simulink model "Feedback_Linearization"  (R2023a)
settings: Solver=ode1be  StartTime=0.0  StopTime=30  FixedStep=0.1  RelTol=1
settings Model: Creator=suhas  LastModifiedBy=suhas
settings SolverCC: ZeroCrossAlgorithm=Adaptive
settings DebuggingCC: IgnoredZcDiagnostic=none

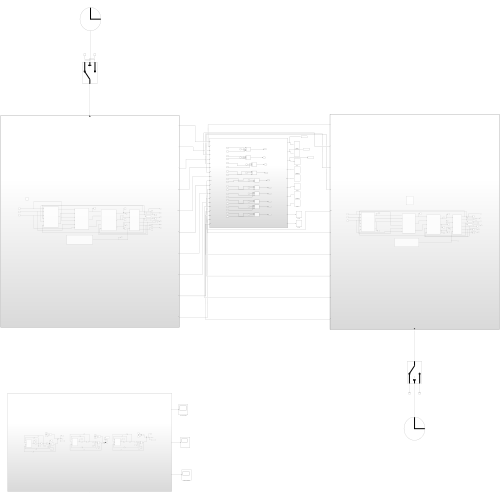
[thumbnail: Simulink's stored preview of the top-level diagram]
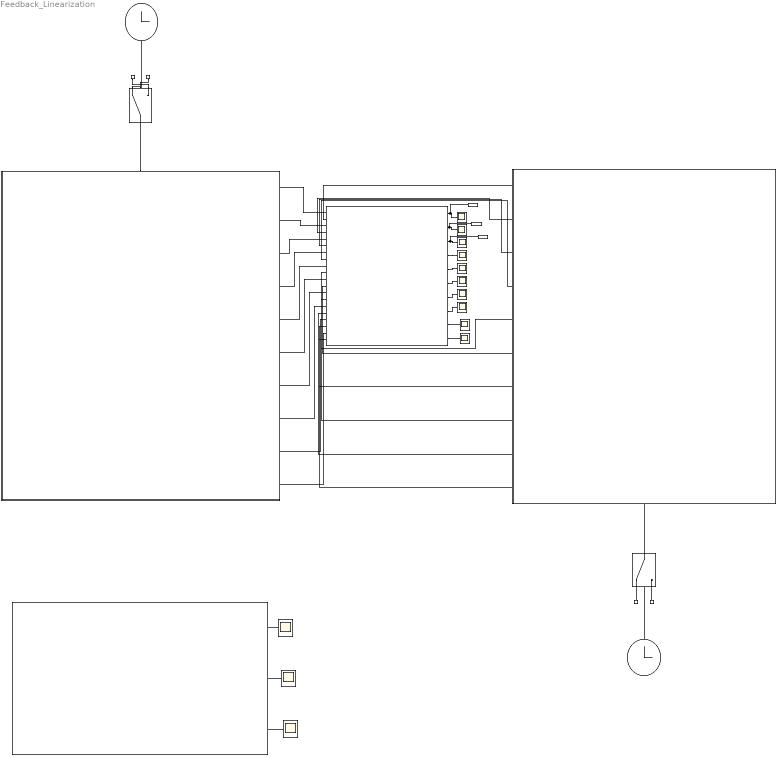
== system Feedback_Linearization ==
  Clock : Clock
  Clock1 : Clock
  Constant : Constant  Value=0
  Constant1 : Constant
  Constant2 : Constant
  Constant3 : Constant  Value=0
  Enabled Subsystem : Subsystem  TreatAsAtomicUnit=on
  Enabled Subsystem1 : Subsystem  TreatAsAtomicUnit=on
  Error Dynamics : Subsystem
  Subsystem : Subsystem
  Switch : Switch  Criteria=u2 > Threshold  Threshold=15  SaturateOnIntegerOverflow=off  InputSameDT=off
  Switch1 : Switch  Criteria=u2 > Threshold  Threshold=15  SaturateOnIntegerOverflow=off  InputSameDT=off
  To Workspace : ToWorkspace  VariableName=x  SaveFormat=Timeseries  SampleTime=-1
  To Workspace1 : ToWorkspace  VariableName=y  SaveFormat=Timeseries  SampleTime=-1
  To Workspace2 : ToWorkspace  VariableName=z  SaveFormat=Timeseries  SampleTime=-1
  X from  Error Dynamics : Scope
  Y from Error Dynamics : Scope
  Z from Error Dynamics : Scope
  phi scope : Scope
  psi scope : Scope
  theta scope : Scope
  u1 scope : Scope
  u2 scope : Scope
  u3 scope : Scope
  u4 scope : Scope
  x scope : Scope
  y scope : Scope
  z scope : Scope
  wires:
  Clock1/1 -> Switch1/2
  Constant3/1 -> Switch1/3
  Clock/1 -> Switch/2
  Constant1/1 -> Switch/3
  Constant2/1 -> Switch1/1
  Constant/1 -> Switch/1
  Switch1/1 -> Enabled Subsystem1/Enable
  Switch/1 -> Enabled Subsystem/Enable
  Enabled Subsystem/1(x) -> Subsystem/1(x1)
  Enabled Subsystem/2(y) -> Subsystem/3(y1)
  Enabled Subsystem/3(z) -> Subsystem/5(z1)
  Enabled Subsystem/4(phi) -> Subsystem/7(phi1)
  Enabled Subsystem/5(theta) -> Subsystem/9(theta1)
  Enabled Subsystem/6(psi) -> Subsystem/11(psi 1)
  Enabled Subsystem/7(u1) -> Subsystem/13(u11)
  Enabled Subsystem/8(u2) -> Subsystem/15(u21)
  Enabled Subsystem/9(u3) -> Subsystem/17(u31)
  Enabled Subsystem/10(u4) -> Subsystem/19(u41)
  Enabled Subsystem1/1(x) -> Subsystem/2(x2)
  Enabled Subsystem1/2(y) -> Subsystem/4(y2)
  Enabled Subsystem1/3(z) -> Subsystem/6(z2)
  Enabled Subsystem1/5(theta) -> Subsystem/10(theta2)
  Enabled Subsystem1/4(phi) -> Subsystem/8(phi2)
  Enabled Subsystem1/6(psi) -> Subsystem/12(psi 2)
  Enabled Subsystem1/8(u1) -> Subsystem/14(u12)
  Enabled Subsystem1/9(u2) -> Subsystem/16(u22)
  Enabled Subsystem1/10(u3) -> Subsystem/18(u32)
  Enabled Subsystem1/7(u4) -> Subsystem/20(u42)
  Subsystem/1(x) -> To Workspace/1, x scope/1
  Subsystem/2(y) -> To Workspace1/1, y scope/1
  Subsystem/3(z) -> To Workspace2/1, z scope/1
  Subsystem/4(phi) -> phi scope/1
  Subsystem/5(theta) -> theta scope/1
  Subsystem/6(psi) -> psi scope/1
  Subsystem/7(u1) -> u1 scope/1
  Subsystem/8(u2) -> u2 scope/1
  Subsystem/9(u3) -> u3 scope/1
  Subsystem/10(u4) -> u4 scope/1
  Error Dynamics/1(x) -> X from  Error Dynamics/1
  Error Dynamics/2(y) -> Y from Error Dynamics/1
  Error Dynamics/3(z) -> Z from Error Dynamics/1

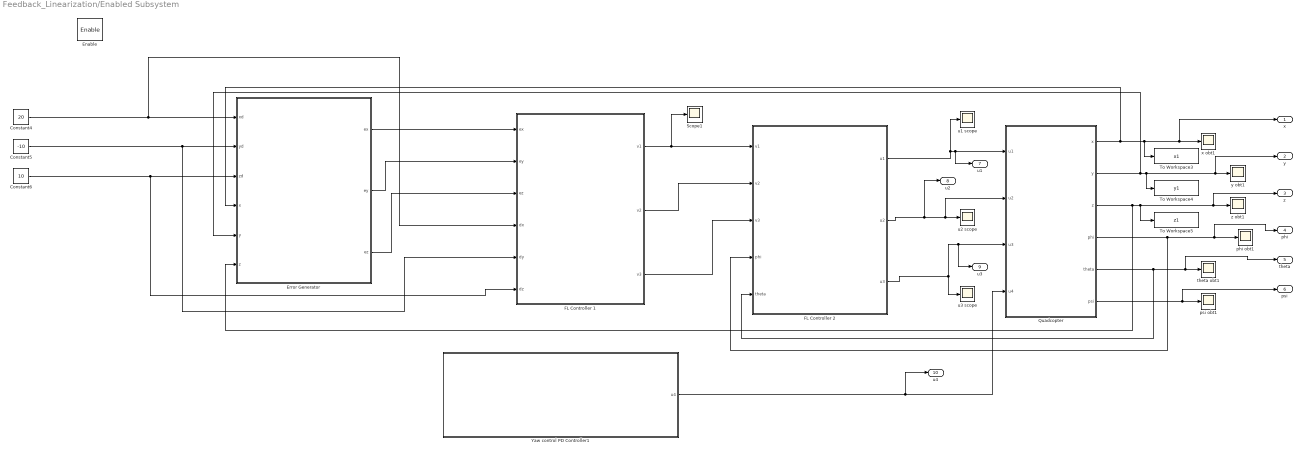
== system Feedback_Linearization/Enabled Subsystem ==
  Enable : EnablePort
  Constant4 : Constant  Value=20
  Constant5 : Constant  Value=-10
  Constant6 : Constant  Value=10
  Error Generator : Subsystem
  FL Controller 1 : Subsystem
  "FL Controller 2 " : Subsystem
  "Quadcopter " : Subsystem
  Scope1 : Scope
  To Workspace3 : ToWorkspace  VariableName=x1  SaveFormat=Timeseries  SampleTime=-1
  To Workspace4 : ToWorkspace  VariableName=y1  SaveFormat=Timeseries  SampleTime=-1
  To Workspace5 : ToWorkspace  VariableName=z1  SaveFormat=Timeseries  SampleTime=-1
  Yaw control PD Controller1 : Subsystem
  phi obt1 : Scope
  psi obt1 : Scope
  theta obt1 : Scope
  u1 scope : Scope
  u2 scope : Scope
  u3 scope : Scope
  x obt1 : Scope
  y obt1 : Scope
  z obt1 : Scope
  x : Outport
  y : Outport  Port=2
  z : Outport  Port=3
  phi : Outport  Port=4
  theta : Outport  Port=5
  psi : Outport  Port=6
  u1 : Outport  Port=7
  u2 : Outport  Port=8
  u3 : Outport  Port=9
  u4 : Outport  Port=10
  wires:
  Error Generator/3(ez) -> FL Controller 1/3(ez)
  "Quadcopter "/1(x) -> Error Generator/4(x), To Workspace3/1, x/1, x obt1/1
  FL Controller 1/2(v2) -> "FL Controller 2 "/2(v2)
  FL Controller 1/1(v1) -> Scope1/1, "FL Controller 2 "/1(v1)
  FL Controller 1/3(v3) -> "FL Controller 2 "/3(v3)
  "Quadcopter "/4(phi) -> "FL Controller 2 "/4(phi), phi/1, phi obt1/1
  "FL Controller 2 "/3(u3) -> u3 scope/1, u3/1, "Quadcopter "/3(u3)
  Error Generator/2(ey) -> FL Controller 1/2(ey)
  Constant4/1 -> FL Controller 1/4(dx), Error Generator/1(xd)
  "Quadcopter "/2(y) -> Error Generator/5(y), To Workspace4/1, y/1, y obt1/1
  "Quadcopter "/6(psi) -> psi/1, psi obt1/1
  Error Generator/1(ex) -> FL Controller 1/1(ex)
  "FL Controller 2 "/1(u1) -> u1 scope/1, u1/1, "Quadcopter "/1(u1)
  Constant6/1 -> FL Controller 1/6(dz), Error Generator/3(zd)
  Yaw control PD Controller1/1(u4) -> u4/1, "Quadcopter "/4(u4)
  Constant5/1 -> FL Controller 1/5(dy), Error Generator/2(yd)
  "FL Controller 2 "/2(u2) -> u2/1, "Quadcopter "/2(u2), u2 scope/1
  "Quadcopter "/5(theta) -> "FL Controller 2 "/5(theta), theta/1, theta obt1/1
  "Quadcopter "/3(z) -> Error Generator/6(z), To Workspace5/1, z/1, z obt1/1

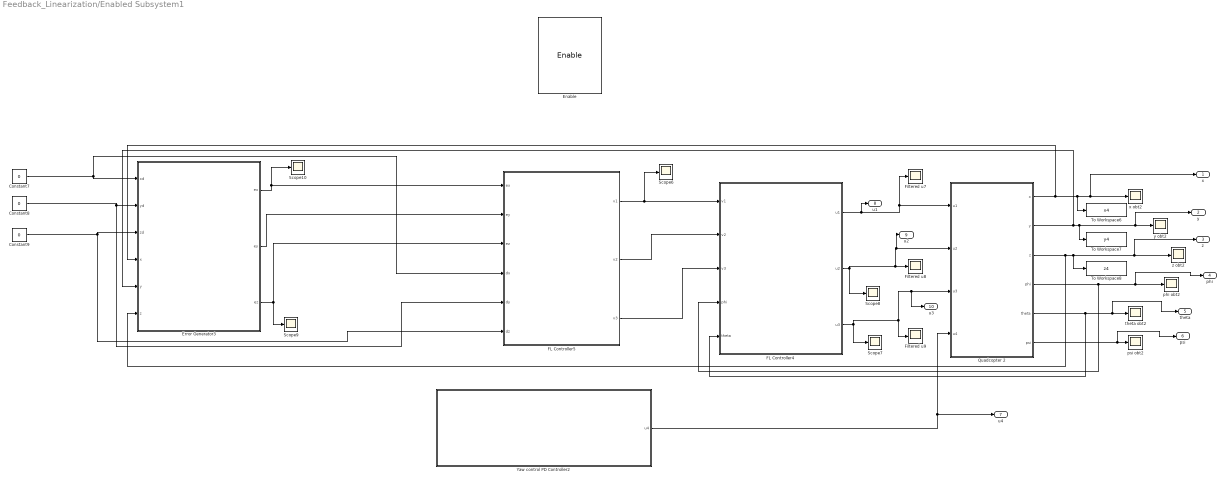
== system Feedback_Linearization/Enabled Subsystem1 ==
  Enable : EnablePort
  Constant7 : Constant  Value=0
  Constant8 : Constant  Value=0
  Constant9 : Constant  Value=0
  Error Generator3 : Subsystem
  FL Controller4 : Subsystem
  FL Controller5 : Subsystem
  Filtered u7 : Scope
  Filtered u8 : Scope
  Filtered u9 : Scope
  Quadcopter 2 : Subsystem
  Scope{6..10} (5 alike) : Scope
  To Workspace6 : ToWorkspace  VariableName=x4  SaveFormat=Timeseries  SampleTime=-1
  To Workspace7 : ToWorkspace  VariableName=y4  SaveFormat=Timeseries  SampleTime=-1
  To Workspace8 : ToWorkspace  VariableName=z4  SaveFormat=Timeseries  SampleTime=-1
  Yaw control PD Controller2 : Subsystem
  phi obt2 : Scope
  psi obt2 : Scope
  theta obt2 : Scope
  x obt2 : Scope
  y obt2 : Scope
  z obt2 : Scope
  x : Outport
  y : Outport  Port=2
  z : Outport  Port=3
  phi : Outport  Port=4
  theta : Outport  Port=5
  psi : Outport  Port=6
  u4 : Outport  Port=7
  u1 : Outport  Port=8
  u2 : Outport  Port=9
  u3 : Outport  Port=10
  wires:
  Quadcopter 2/1(x) -> Error Generator3/4(x), To Workspace6/1, x/1, x obt2/1
  FL Controller5/3(v3) -> FL Controller4/3(v3)
  Quadcopter 2/3(z) -> Error Generator3/6(z), To Workspace8/1, z obt2/1, z/1
  Quadcopter 2/4(phi) -> FL Controller4/4(phi), phi/1, phi obt2/1
  Constant8/1 -> FL Controller5/5(dy), Error Generator3/2(yd)
  Quadcopter 2/5(theta) -> FL Controller4/5(theta), theta/1, theta obt2/1
  FL Controller5/1(v1) -> Scope6/1, FL Controller4/1(v1)
  FL Controller4/3(u3) -> Filtered u9/1, u3/1, Quadcopter 2/3(u3), Scope7/1
  Constant7/1 -> FL Controller5/4(dx), Error Generator3/1(xd)
  Error Generator3/2(ey) -> FL Controller5/2(ey)
  FL Controller4/1(u1) -> u1/1, Filtered u7/1, Quadcopter 2/1(u1)
  FL Controller5/2(v2) -> FL Controller4/2(v2)
  Error Generator3/1(ex) -> Scope10/1, FL Controller5/1(ex)
  Error Generator3/3(ez) -> FL Controller5/3(ez), Scope9/1
  Yaw control PD Controller2/1(u4) -> u4/1, Quadcopter 2/4(u4)
  Constant9/1 -> Error Generator3/3(zd), FL Controller5/6(dz)
  Quadcopter 2/6(psi) -> psi/1, psi obt2/1
  Quadcopter 2/2(y) -> Error Generator3/5(y), To Workspace7/1, y/1, y obt2/1
  FL Controller4/2(u2) -> u2/1, Quadcopter 2/2(u2), Filtered u8/1, Scope8/1

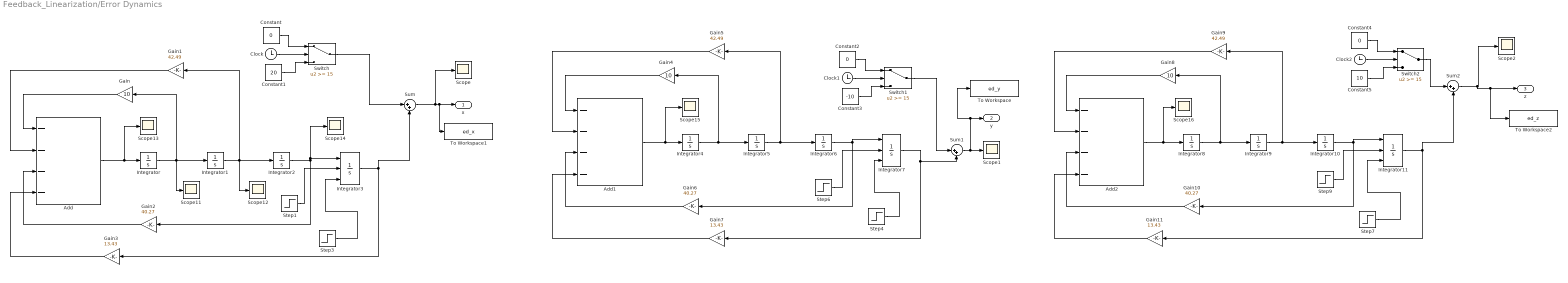
== system Feedback_Linearization/Error Dynamics ==
  Add : Sum  Inputs=----
  Add1 : Sum  Inputs=----
  Add2 : Sum  Inputs=----
  Clock : Clock
  Clock1 : Clock
  Clock2 : Clock
  Constant : Constant  Value=0
  Constant1 : Constant  Value=20
  Constant2 : Constant  Value=0
  Constant3 : Constant  Value=-10
  Constant4 : Constant  Value=0
  Constant5 : Constant  Value=10
  Gain : Gain  Gain=10
  Gain1 : Gain  Gain=42.49
  Gain10 : Gain  Gain=40.27
  Gain11 : Gain  Gain=13.43
  Gain2 : Gain  Gain=40.27
  Gain3 : Gain  Gain=13.43
  Gain4 : Gain  Gain=10
  Gain5 : Gain  Gain=42.49
  Gain6 : Gain  Gain=40.27
  Gain7 : Gain  Gain=13.43
  Gain8 : Gain  Gain=10
  Gain9 : Gain  Gain=42.49
  Integrator{,1..2,4..6,8..10} (9 alike) : Integrator
  Integrator11 : Integrator  ExternalReset=rising  InitialConditionSource=external
  Integrator3 : Integrator  ExternalReset=rising  InitialConditionSource=external
  Integrator7 : Integrator  ExternalReset=rising  InitialConditionSource=external
  Scope{,1..2,11..16} (9 alike) : Scope
  Step1 : Step  Time=15  SampleTime=0
  Step3 : Step  Time=15  Before=-10  After=20  SampleTime=0
  Step4 : Step  Time=15  Before=20  After=-10  SampleTime=0
  Step6 : Step  Time=15  SampleTime=0
  Step7 : Step  Time=15  Before=10  After=10  SampleTime=0
  Step9 : Step  Time=15  SampleTime=0
  Sum : Sum  Inputs=|++
  Sum1 : Sum  Inputs=|++
  Sum2 : Sum  Inputs=|++
  Switch : Switch  Threshold=15  SaturateOnIntegerOverflow=off  InputSameDT=off
  Switch1 : Switch  Threshold=15  SaturateOnIntegerOverflow=off  InputSameDT=off
  Switch2 : Switch  Threshold=15  SaturateOnIntegerOverflow=off  InputSameDT=off
  To Workspace : ToWorkspace  VariableName=ed_y  SaveFormat=Timeseries  SampleTime=-1
  To Workspace1 : ToWorkspace  VariableName=ed_x  SaveFormat=Timeseries  SampleTime=-1
  To Workspace2 : ToWorkspace  VariableName=ed_z  SaveFormat=Timeseries  SampleTime=-1
  x : Outport
  y : Outport  Port=2
  z : Outport  Port=3
  wires:
  Integrator/1 -> Scope11/1, Gain/1, Integrator1/1
  Integrator1/1 -> Scope12/1, Gain1/1, Integrator2/1
  Integrator2/1 -> Scope14/1, Integrator3/1, Gain2/1
  Integrator3/1 -> Sum/2, Gain3/1
  Gain/1 -> Add/1
  Gain1/1 -> Add/2
  Gain2/1 -> Add/3
  Gain3/1 -> Add/4
  Step3/1 -> Integrator3/3
  Switch/1 -> Sum/1
  Sum/1 -> To Workspace1/1, x/1, Scope/1
  Switch1/1 -> Sum1/1
  Gain5/1 -> Add1/2
  Gain4/1 -> Add1/1
  Sum1/1 -> To Workspace/1, y/1, Scope1/1
  Gain7/1 -> Add1/4
  Gain6/1 -> Add1/3
  Switch2/1 -> Sum2/1
  Gain9/1 -> Add2/2
  Gain8/1 -> Add2/1
  Integrator9/1 -> Gain9/1, Integrator10/1
  Gain11/1 -> Add2/4
  Integrator10/1 -> Gain10/1, Integrator11/1
  Gain10/1 -> Add2/3
  Sum2/1 -> To Workspace2/1, z/1, Scope2/1
  Add/1 -> Scope13/1, Integrator/1
  Add1/1 -> Scope15/1, Integrator4/1
  Step4/1 -> Integrator7/3
  Step7/1 -> Integrator11/3
  Add2/1 -> Scope16/1, Integrator8/1
  Step9/1 -> Integrator11/2
  Step6/1 -> Integrator7/2
  Step1/1 -> Integrator3/2
  Integrator7/1 -> Gain7/1, Sum1/2
  Integrator6/1 -> Gain6/1, Integrator7/1
  Integrator5/1 -> Gain5/1, Integrator6/1
  Integrator4/1 -> Gain4/1, Integrator5/1
  Integrator8/1 -> Gain8/1, Integrator9/1
  Integrator11/1 -> Sum2/2, Gain11/1
  Clock/1 -> Switch/2
  Constant/1 -> Switch/1
  Constant1/1 -> Switch/3
  Constant2/1 -> Switch1/1
  Constant3/1 -> Switch1/3
  Clock1/1 -> Switch1/2
  Constant4/1 -> Switch2/1
  Constant5/1 -> Switch2/3
  Clock2/1 -> Switch2/2

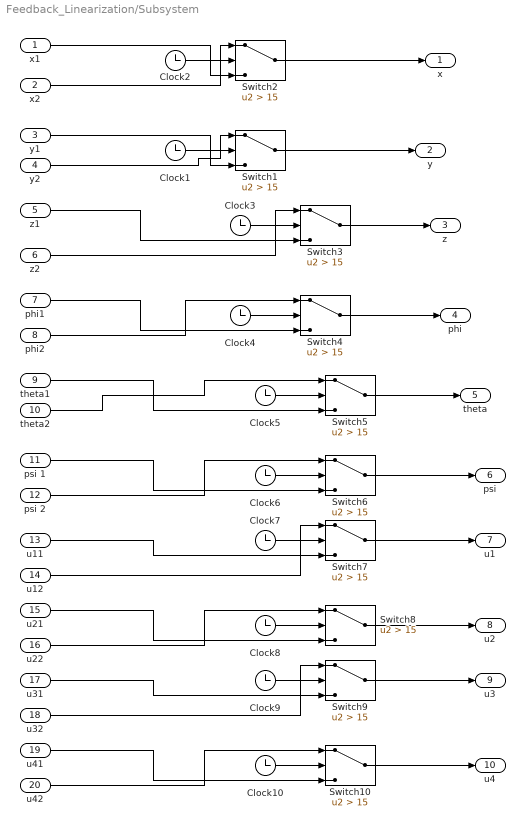
== system Feedback_Linearization/Subsystem ==
  x1 : Inport
  x2 : Inport  Port=2
  y1 : Inport  Port=3
  y2 : Inport  Port=4
  z1 : Inport  Port=5
  z2 : Inport  Port=6
  phi1 : Inport  Port=7
  phi2 : Inport  Port=8
  theta1 : Inport  Port=9
  theta2 : Inport  Port=10
  psi 1 : Inport  Port=11
  psi 2 : Inport  Port=12
  u11 : Inport  Port=13
  u12 : Inport  Port=14
  u21 : Inport  Port=15
  u22 : Inport  Port=16
  u31 : Inport  Port=17
  u32 : Inport  Port=18
  u41 : Inport  Port=19
  u42 : Inport  Port=20
  Clock{1..10} (10 alike) : Clock
  Switch{1..10} (10 alike) : Switch  Criteria=u2 > Threshold  Threshold=15  SaturateOnIntegerOverflow=off  InputSameDT=off
  x : Outport
  y : Outport  Port=2
  z : Outport  Port=3
  phi : Outport  Port=4
  theta : Outport  Port=5
  psi : Outport  Port=6
  u1 : Outport  Port=7
  u2 : Outport  Port=8
  u3 : Outport  Port=9
  u4 : Outport  Port=10
  wires:
  Clock2/1 -> Switch2/2
  x1/1 -> Switch2/3
  x2/1 -> Switch2/1
  y2/1 -> Switch1/1
  Clock1/1 -> Switch1/2
  y1/1 -> Switch1/3
  z2/1 -> Switch3/1
  Clock3/1 -> Switch3/2
  z1/1 -> Switch3/3
  phi2/1 -> Switch4/1
  Clock4/1 -> Switch4/2
  phi1/1 -> Switch4/3
  theta2/1 -> Switch5/1
  Clock5/1 -> Switch5/2
  theta1/1 -> Switch5/3
  psi 2/1 -> Switch6/1
  Clock6/1 -> Switch6/2
  psi 1/1 -> Switch6/3
  u12/1 -> Switch7/1
  Clock7/1 -> Switch7/2
  u11/1 -> Switch7/3
  u22/1 -> Switch8/1
  Clock8/1 -> Switch8/2
  u21/1 -> Switch8/3
  u32/1 -> Switch9/1
  Clock9/1 -> Switch9/2
  u31/1 -> Switch9/3
  u42/1 -> Switch10/1
  Clock10/1 -> Switch10/2
  u41/1 -> Switch10/3
  Switch2/1 -> x/1
  Switch1/1 -> y/1
  Switch3/1 -> z/1
  Switch4/1 -> phi/1
  Switch5/1 -> theta/1
  Switch6/1 -> psi/1
  Switch7/1 -> u1/1
  Switch8/1 -> u2/1
  Switch9/1 -> u3/1
  Switch10/1 -> u4/1

== system Feedback_Linearization/Enabled Subsystem/Error Generator ==
  xd : Inport
  yd : Inport  Port=2
  zd : Inport  Port=3
  x : Inport  Port=4
  y : Inport  Port=5
  z : Inport  Port=6
  Subtract : Sum  Inputs=+-
  Subtract1 : Sum  Inputs=+-
  Subtract2 : Sum  Inputs=+-
  ex : Outport
  ey : Outport  Port=2
  ez : Outport  Port=3
  wires:
  xd/1 -> Subtract/2
  x/1 -> Subtract/1
  Subtract/1 -> ex/1
  yd/1 -> Subtract1/2
  y/1 -> Subtract1/1
  z/1 -> Subtract2/1
  zd/1 -> Subtract2/2
  Subtract1/1 -> ey/1
  Subtract2/1 -> ez/1

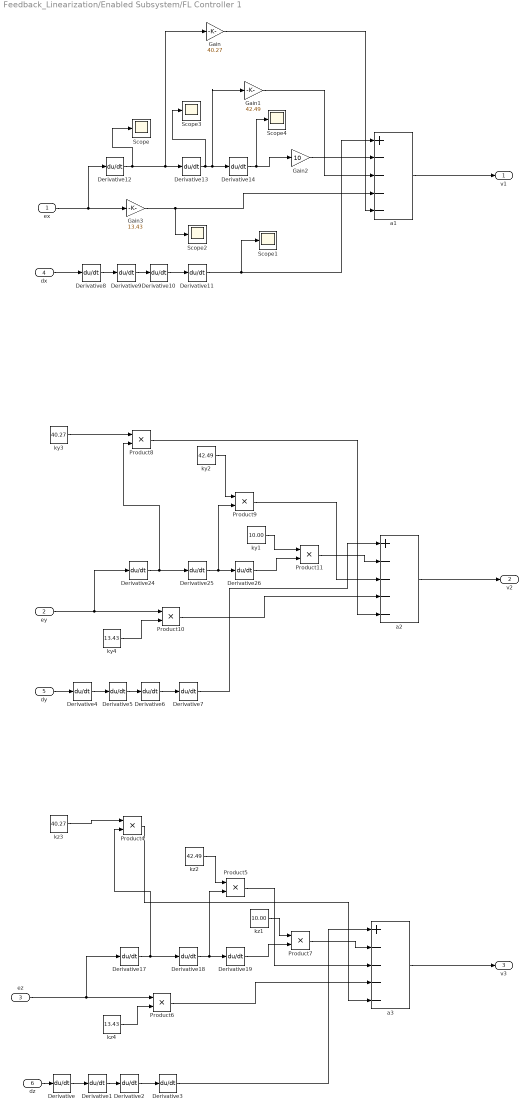
== system Feedback_Linearization/Enabled Subsystem/FL Controller 1 ==
  ex : Inport
  ey : Inport  Port=2
  ez : Inport  Port=3
  dx : Inport  Port=4
  dy : Inport  Port=5
  dz : Inport  Port=6
  Derivative{,1..14,17..19,24..26} (21 alike) : Derivative
  Gain : Gain  Gain=40.27
  Gain1 : Gain  Gain=42.49
  Gain2 : Gain  Gain=10
  Gain3 : Gain  Gain=13.43
  Product{4..11} (8 alike) : Product
  Scope{,1..4} (5 alike) : Scope
  a1 : Sum  Inputs=+----
  a2 : Sum  Inputs=+----
  a3 : Sum  Inputs=+----
  ky1 : Constant  Value=10.00
  ky2 : Constant  Value=42.49
  ky3 : Constant  Value=40.27
  ky4 : Constant  Value=13.43
  kz1 : Constant  Value=10.00
  kz2 : Constant  Value=42.49
  kz3 : Constant  Value=40.27
  kz4 : Constant  Value=13.43
  v1 : Outport
  v2 : Outport  Port=2
  v3 : Outport  Port=3
  wires:
  ex/1 -> Gain3/1, Derivative12/1
  Derivative12/1 -> Scope/1, Derivative13/1, Gain/1
  Derivative13/1 -> Scope3/1, Gain1/1, Derivative14/1
  Derivative14/1 -> Scope4/1, Gain2/1
  Gain3/1 -> Scope2/1, a1/4
  a1/1 -> v1/1
  a3/1 -> v3/1
  kz1/1 -> Product7/1
  Derivative17/1 -> Product4/2, Derivative18/1
  Derivative18/1 -> Product5/2, Derivative19/1
  Product6/1 -> a3/4
  Product4/1 -> a3/5
  Product7/1 -> a3/2
  Product5/1 -> a3/3
  kz4/1 -> Product6/2
  kz2/1 -> Product5/1
  kz3/1 -> Product4/1
  ez/1 -> Product6/1, Derivative17/1
  Derivative19/1 -> Product7/2
  a2/1 -> v2/1
  Derivative24/1 -> Product8/2, Derivative25/1
  Derivative25/1 -> Product9/2, Derivative26/1
  Product10/1 -> a2/4
  Product8/1 -> a2/5
  Product11/1 -> a2/2
  Product9/1 -> a2/3
  ey/1 -> Product10/1, Derivative24/1
  Derivative26/1 -> Product11/2
  ky3/1 -> Product8/1
  ky2/1 -> Product9/1
  ky1/1 -> Product11/1
  ky4/1 -> Product10/2
  dz/1 -> Derivative/1
  Derivative/1 -> Derivative1/1
  Derivative1/1 -> Derivative2/1
  Derivative2/1 -> Derivative3/1
  Derivative6/1 -> Derivative7/1
  Derivative5/1 -> Derivative6/1
  Derivative4/1 -> Derivative5/1
  dy/1 -> Derivative4/1
  Derivative10/1 -> Derivative11/1
  Derivative9/1 -> Derivative10/1
  Derivative8/1 -> Derivative9/1
  dx/1 -> Derivative8/1
  Gain/1 -> a1/5
  Gain1/1 -> a1/3
  Gain2/1 -> a1/2
  Derivative11/1 -> a1/1, Scope1/1
  Derivative7/1 -> a2/1
  Derivative3/1 -> a3/1

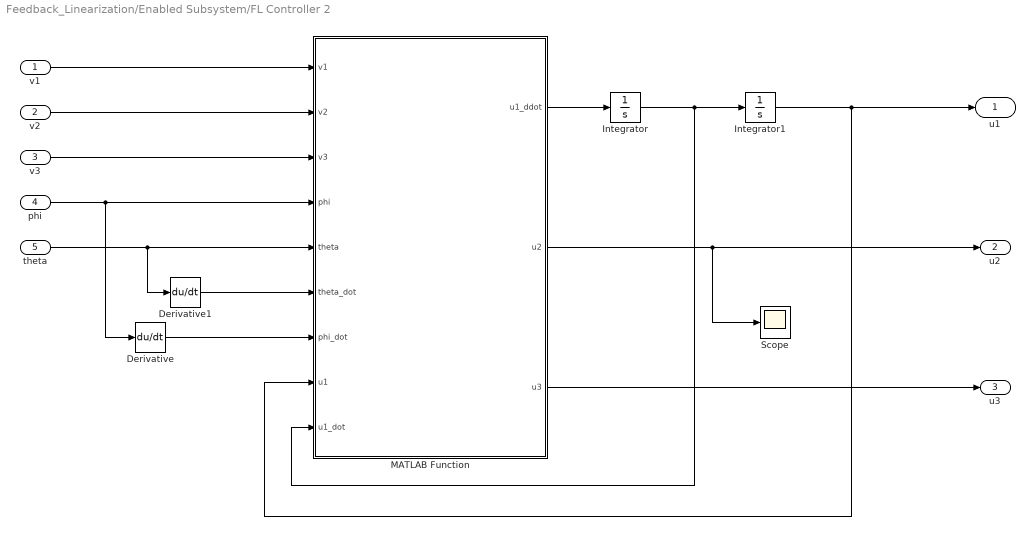
== system Feedback_Linearization/Enabled Subsystem/FL Controller 2  ==
  v1 : Inport
  v2 : Inport  Port=2
  v3 : Inport  Port=3
  phi : Inport  Port=4
  theta : Inport  Port=5
  Derivative : Derivative
  Derivative1 : Derivative
  Integrator : Integrator
  Integrator1 : Integrator  InitialCondition=9.81  UpperSaturationLimit=15  LowerSaturationLimit=0
  MATLAB Function : MATLAB Function  TreatAsAtomicUnit=on
  Scope : Scope
  u1 : Outport
  u2 : Outport  Port=2
  u3 : Outport  Port=3
  wires:
  v1/1 -> MATLAB Function/1(v1)
  v3/1 -> MATLAB Function/3(v3)
  v2/1 -> MATLAB Function/2(v2)
  MATLAB Function/1(u1_ddot) -> Integrator/1
  MATLAB Function/2(u2) -> Scope/1, u2/1
  MATLAB Function/3(u3) -> u3/1
  phi/1 -> Derivative/1, MATLAB Function/4(phi)
  theta/1 -> Derivative1/1, MATLAB Function/5(theta)
  Derivative/1 -> MATLAB Function/7(phi_dot)
  Derivative1/1 -> MATLAB Function/6(theta_dot)
  Integrator1/1 -> MATLAB Function/8(u1), u1/1
  Integrator/1 -> MATLAB Function/9(u1_dot), Integrator1/1

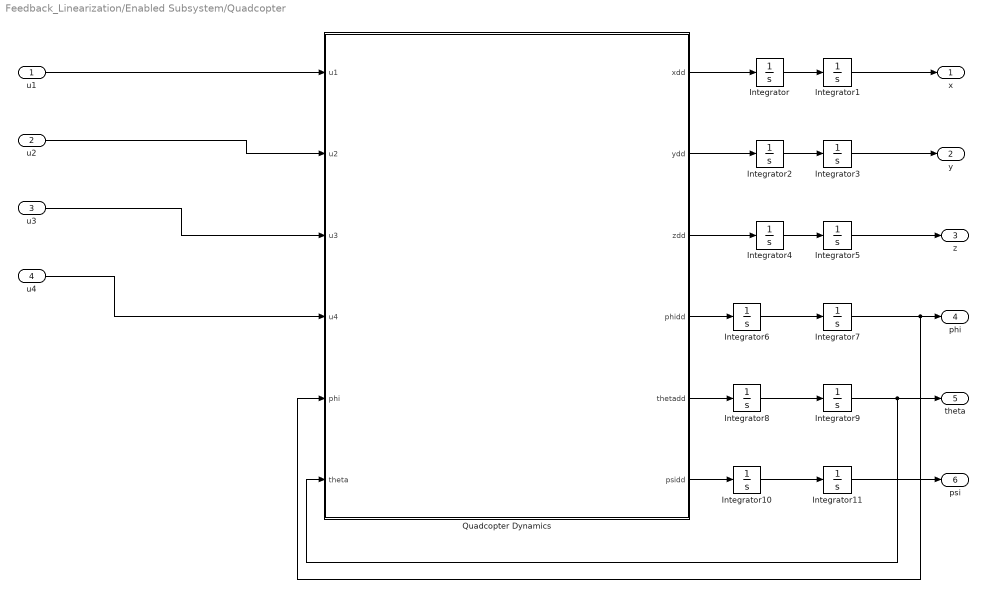
== system Feedback_Linearization/Enabled Subsystem/Quadcopter  ==
  u1 : Inport
  u2 : Inport  Port=2
  u3 : Inport  Port=3
  u4 : Inport  Port=4
  Integrator{,2,4,10} (4 alike) : Integrator
  Integrator1 : Integrator  InitialCondition=10
  Integrator11 : Integrator  InitialCondition=0.5235
  Integrator3 : Integrator  InitialCondition=10
  Integrator5 : Integrator  InitialCondition=20
  Integrator6 : Integrator  UpperSaturationLimit=0.1  LowerSaturationLimit=-0.1
  Integrator7 : Integrator  InitialCondition=0.5325
  Integrator8 : Integrator  UpperSaturationLimit=0.1  LowerSaturationLimit=-0.1
  Integrator9 : Integrator  InitialCondition=0.5325
  Quadcopter Dynamics : MATLAB Function  TreatAsAtomicUnit=on
  x : Outport
  y : Outport  Port=2
  z : Outport  Port=3
  phi : Outport  Port=4
  theta : Outport  Port=5
  psi : Outport  Port=6
  wires:
  u1/1 -> Quadcopter Dynamics/1(u1)
  u2/1 -> Quadcopter Dynamics/2(u2)
  u3/1 -> Quadcopter Dynamics/3(u3)
  u4/1 -> Quadcopter Dynamics/4(u4)
  Quadcopter Dynamics/1(xdd) -> Integrator/1
  Quadcopter Dynamics/2(ydd) -> Integrator2/1
  Quadcopter Dynamics/3(zdd) -> Integrator4/1
  Quadcopter Dynamics/4(phidd) -> Integrator6/1
  Quadcopter Dynamics/5(thetadd) -> Integrator8/1
  Quadcopter Dynamics/6(psidd) -> Integrator10/1
  Integrator/1 -> Integrator1/1
  Integrator2/1 -> Integrator3/1
  Integrator4/1 -> Integrator5/1
  Integrator6/1 -> Integrator7/1
  Integrator8/1 -> Integrator9/1
  Integrator10/1 -> Integrator11/1
  Integrator1/1 -> x/1
  Integrator3/1 -> y/1
  Integrator5/1 -> z/1
  Integrator7/1 -> phi/1, Quadcopter Dynamics/5(phi)
  Integrator9/1 -> theta/1, Quadcopter Dynamics/6(theta)
  Integrator11/1 -> psi/1

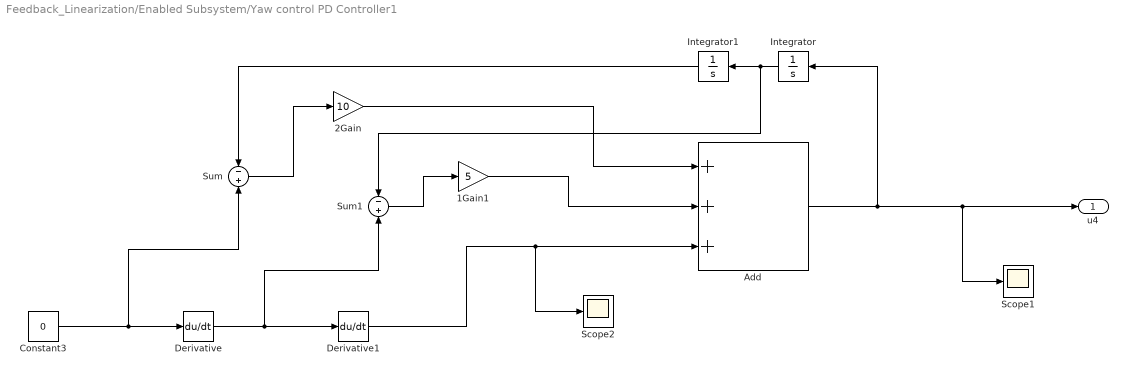
== system Feedback_Linearization/Enabled Subsystem/Yaw control PD Controller1 ==
  1Gain1 : Gain  Gain=5
  2Gain : Gain  Gain=10
  Add : Sum  Inputs=+++
  Constant3 : Constant  Value=0
  Derivative : Derivative
  Derivative1 : Derivative
  Integrator : Integrator
  Integrator1 : Integrator  InitialCondition=0.5235
  Scope1 : Scope
  Scope2 : Scope
  Sum : Sum  Inputs=-+
  Sum1 : Sum  Inputs=-+
  u4 : Outport
  wires:
  Derivative/1 -> Sum1/2, Derivative1/1
  Sum/1 -> 2Gain/1
  Derivative1/1 -> Scope2/1, Add/3
  Constant3/1 -> Sum/2, Derivative/1
  Sum1/1 -> 1Gain1/1
  1Gain1/1 -> Add/2
  2Gain/1 -> Add/1
  Add/1 -> u4/1, Scope1/1, Integrator/1
  Integrator/1 -> Sum1/1, Integrator1/1
  Integrator1/1 -> Sum/1

== system Feedback_Linearization/Enabled Subsystem1/Error Generator3 ==
  xd : Inport
  yd : Inport  Port=2
  zd : Inport  Port=3
  x : Inport  Port=4
  y : Inport  Port=5
  z : Inport  Port=6
  Subtract : Sum  Inputs=+-
  Subtract1 : Sum  Inputs=+-
  Subtract2 : Sum  Inputs=+-
  ex : Outport
  ey : Outport  Port=2
  ez : Outport  Port=3
  wires:
  xd/1 -> Subtract/2
  x/1 -> Subtract/1
  Subtract/1 -> ex/1
  yd/1 -> Subtract1/2
  y/1 -> Subtract1/1
  z/1 -> Subtract2/1
  zd/1 -> Subtract2/2
  Subtract1/1 -> ey/1
  Subtract2/1 -> ez/1

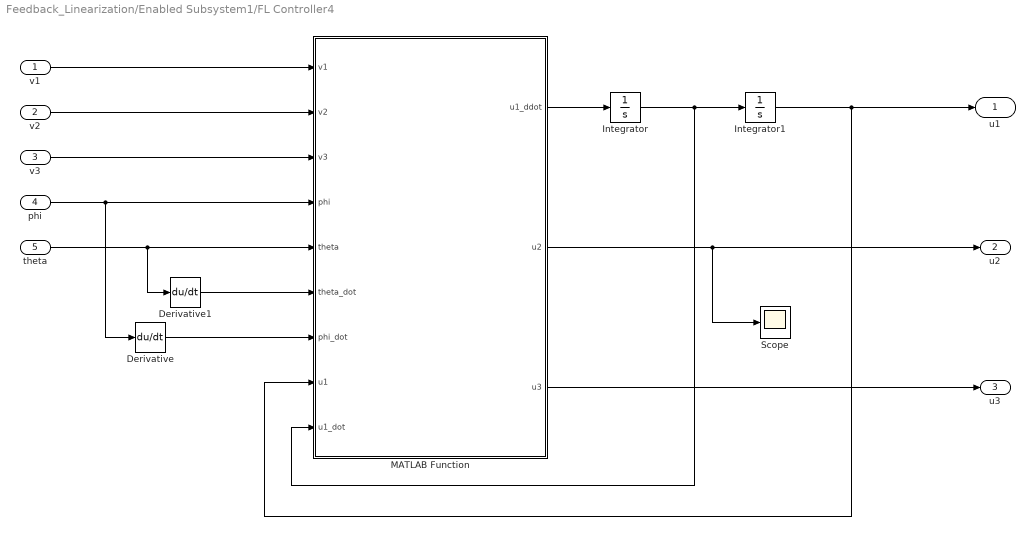
== system Feedback_Linearization/Enabled Subsystem1/FL Controller4 ==
  v1 : Inport
  v2 : Inport  Port=2
  v3 : Inport  Port=3
  phi : Inport  Port=4
  theta : Inport  Port=5
  Derivative : Derivative
  Derivative1 : Derivative
  Integrator : Integrator
  Integrator1 : Integrator  InitialCondition=9.81  UpperSaturationLimit=15  LowerSaturationLimit=0
  MATLAB Function : MATLAB Function  TreatAsAtomicUnit=on
  Scope : Scope
  u1 : Outport
  u2 : Outport  Port=2
  u3 : Outport  Port=3
  wires:
  v1/1 -> MATLAB Function/1(v1)
  v3/1 -> MATLAB Function/3(v3)
  v2/1 -> MATLAB Function/2(v2)
  MATLAB Function/1(u1_ddot) -> Integrator/1
  MATLAB Function/2(u2) -> Scope/1, u2/1
  MATLAB Function/3(u3) -> u3/1
  phi/1 -> Derivative/1, MATLAB Function/4(phi)
  theta/1 -> Derivative1/1, MATLAB Function/5(theta)
  Derivative/1 -> MATLAB Function/7(phi_dot)
  Derivative1/1 -> MATLAB Function/6(theta_dot)
  Integrator1/1 -> MATLAB Function/8(u1), u1/1
  Integrator/1 -> MATLAB Function/9(u1_dot), Integrator1/1

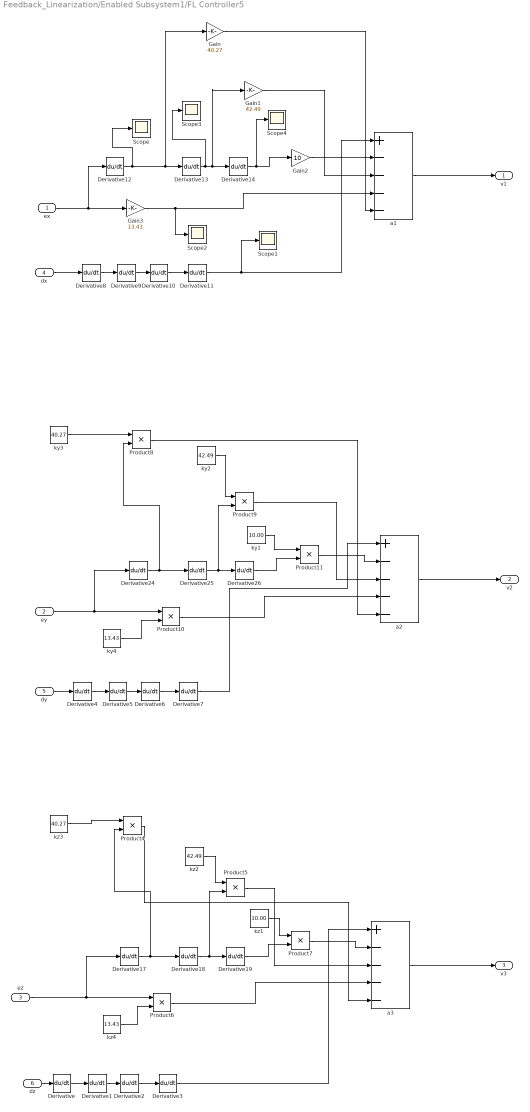
== system Feedback_Linearization/Enabled Subsystem1/FL Controller5 ==
  ex : Inport
  ey : Inport  Port=2
  ez : Inport  Port=3
  dx : Inport  Port=4
  dy : Inport  Port=5
  dz : Inport  Port=6
  Derivative{,1..14,17..19,24..26} (21 alike) : Derivative
  Gain : Gain  Gain=40.27
  Gain1 : Gain  Gain=42.49
  Gain2 : Gain  Gain=10
  Gain3 : Gain  Gain=13.43
  Product{4..11} (8 alike) : Product
  Scope{,1..4} (5 alike) : Scope
  a1 : Sum  Inputs=+----
  a2 : Sum  Inputs=+----
  a3 : Sum  Inputs=+----
  ky1 : Constant  Value=10.00
  ky2 : Constant  Value=42.49
  ky3 : Constant  Value=40.27
  ky4 : Constant  Value=13.43
  kz1 : Constant  Value=10.00
  kz2 : Constant  Value=42.49
  kz3 : Constant  Value=40.27
  kz4 : Constant  Value=13.43
  v1 : Outport
  v2 : Outport  Port=2
  v3 : Outport  Port=3
  wires:
  ex/1 -> Gain3/1, Derivative12/1
  Derivative12/1 -> Scope/1, Derivative13/1, Gain/1
  Derivative13/1 -> Scope3/1, Gain1/1, Derivative14/1
  Derivative14/1 -> Scope4/1, Gain2/1
  Gain3/1 -> Scope2/1, a1/4
  a1/1 -> v1/1
  a3/1 -> v3/1
  kz1/1 -> Product7/1
  Derivative17/1 -> Product4/2, Derivative18/1
  Derivative18/1 -> Product5/2, Derivative19/1
  Product6/1 -> a3/4
  Product4/1 -> a3/5
  Product7/1 -> a3/2
  Product5/1 -> a3/3
  kz4/1 -> Product6/2
  kz2/1 -> Product5/1
  kz3/1 -> Product4/1
  ez/1 -> Product6/1, Derivative17/1
  Derivative19/1 -> Product7/2
  a2/1 -> v2/1
  Derivative24/1 -> Product8/2, Derivative25/1
  Derivative25/1 -> Product9/2, Derivative26/1
  Product10/1 -> a2/4
  Product8/1 -> a2/5
  Product11/1 -> a2/2
  Product9/1 -> a2/3
  ey/1 -> Product10/1, Derivative24/1
  Derivative26/1 -> Product11/2
  ky3/1 -> Product8/1
  ky2/1 -> Product9/1
  ky1/1 -> Product11/1
  ky4/1 -> Product10/2
  dz/1 -> Derivative/1
  Derivative/1 -> Derivative1/1
  Derivative1/1 -> Derivative2/1
  Derivative2/1 -> Derivative3/1
  Derivative6/1 -> Derivative7/1
  Derivative5/1 -> Derivative6/1
  Derivative4/1 -> Derivative5/1
  dy/1 -> Derivative4/1
  Derivative10/1 -> Derivative11/1
  Derivative9/1 -> Derivative10/1
  Derivative8/1 -> Derivative9/1
  dx/1 -> Derivative8/1
  Gain/1 -> a1/5
  Gain1/1 -> a1/3
  Gain2/1 -> a1/2
  Derivative11/1 -> a1/1, Scope1/1
  Derivative7/1 -> a2/1
  Derivative3/1 -> a3/1

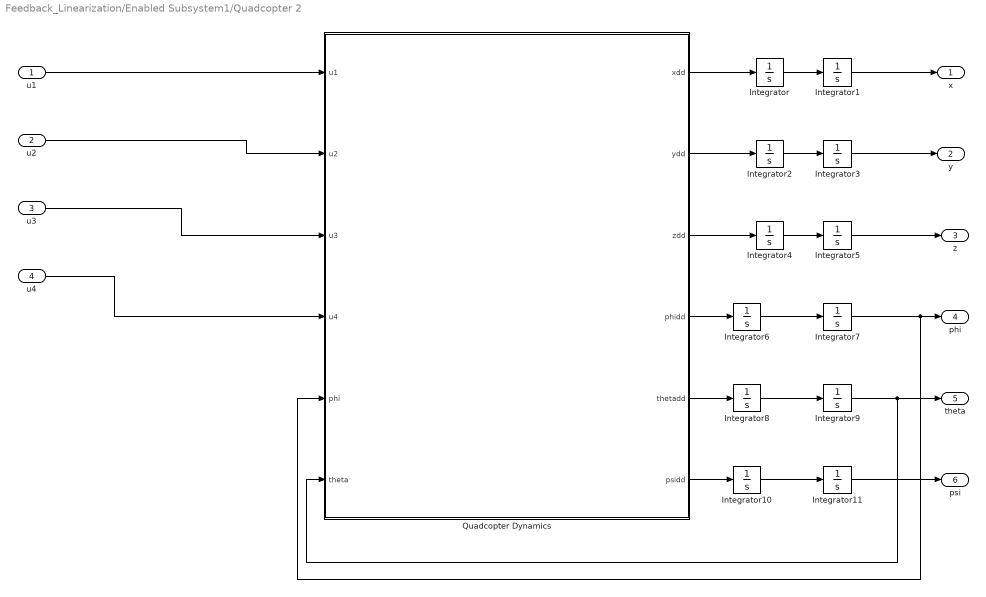
== system Feedback_Linearization/Enabled Subsystem1/Quadcopter 2 ==
  u1 : Inport
  u2 : Inport  Port=2
  u3 : Inport  Port=3
  u4 : Inport  Port=4
  Integrator{,2,4,7,9..11} (7 alike) : Integrator
  Integrator1 : Integrator  InitialCondition=20
  Integrator3 : Integrator  InitialCondition=-10
  Integrator5 : Integrator  InitialCondition=10
  Integrator6 : Integrator  UpperSaturationLimit=0.1  LowerSaturationLimit=-0.1
  Integrator8 : Integrator  UpperSaturationLimit=0.1  LowerSaturationLimit=-0.1
  Quadcopter Dynamics : MATLAB Function  TreatAsAtomicUnit=on
  x : Outport
  y : Outport  Port=2
  z : Outport  Port=3
  phi : Outport  Port=4
  theta : Outport  Port=5
  psi : Outport  Port=6
  wires:
  u1/1 -> Quadcopter Dynamics/1(u1)
  u2/1 -> Quadcopter Dynamics/2(u2)
  u3/1 -> Quadcopter Dynamics/3(u3)
  u4/1 -> Quadcopter Dynamics/4(u4)
  Quadcopter Dynamics/1(xdd) -> Integrator/1
  Quadcopter Dynamics/2(ydd) -> Integrator2/1
  Quadcopter Dynamics/3(zdd) -> Integrator4/1
  Quadcopter Dynamics/4(phidd) -> Integrator6/1
  Quadcopter Dynamics/5(thetadd) -> Integrator8/1
  Quadcopter Dynamics/6(psidd) -> Integrator10/1
  Integrator/1 -> Integrator1/1
  Integrator2/1 -> Integrator3/1
  Integrator4/1 -> Integrator5/1
  Integrator6/1 -> Integrator7/1
  Integrator8/1 -> Integrator9/1
  Integrator10/1 -> Integrator11/1
  Integrator1/1 -> x/1
  Integrator3/1 -> y/1
  Integrator5/1 -> z/1
  Integrator7/1 -> phi/1, Quadcopter Dynamics/5(phi)
  Integrator9/1 -> theta/1, Quadcopter Dynamics/6(theta)
  Integrator11/1 -> psi/1

== system Feedback_Linearization/Enabled Subsystem1/Yaw control PD Controller2 ==
  1Gain1 : Gain  Gain=5
  2Gain : Gain  Gain=10
  Add : Sum  Inputs=+++
  Constant3 : Constant  Value=0
  Derivative : Derivative
  Derivative1 : Derivative
  Integrator : Integrator
  Integrator1 : Integrator
  Scope1 : Scope
  Scope2 : Scope
  Sum : Sum  Inputs=-+
  Sum1 : Sum  Inputs=-+
  u4 : Outport
  wires:
  Derivative/1 -> Sum1/2, Derivative1/1
  Sum/1 -> 2Gain/1
  Derivative1/1 -> Scope2/1, Add/3
  Constant3/1 -> Sum/2, Derivative/1
  Sum1/1 -> 1Gain1/1
  1Gain1/1 -> Add/2
  2Gain/1 -> Add/1
  Add/1 -> u4/1, Scope1/1, Integrator/1
  Integrator/1 -> Sum1/1, Integrator1/1
  Integrator1/1 -> Sum/1

== matlab function Feedback_Linearization/Enabled Subsystem/FL Controller 2 /MATLAB Function ==
  data: v1 input; u1_ddot output; v2 input; v3 input; phi input; theta input; theta_dot input; phi_dot input; u1 input; u1_dot input; u2 output; u3 output
function [u1_ddot,u2,u3] = fcn(v1,v2,v3,phi,theta,theta_dot,phi_dot,u1,u1_dot)

m1=[[sin(theta),0,(u1)*cos(theta)];
    [-sin(phi),(-u1*cos(phi)),0];
    [(cos(theta)*cos(phi)),(-u1*cos(theta)*sin(phi)),(-u1*sin(theta)*cos(phi))]];


m2=[(-2*u1_dot*theta_dot*cos(theta))+(u1*((theta_dot*theta_dot))*sin(theta))+v1;
    (2*u1_dot*phi_dot*cos(phi))-(u1*((phi_dot*phi_dot))*sin(phi))+v2;
    (2*u1_dot*theta_dot*sin(theta)*cos(phi))+(2*u1_dot*phi_dot*cos(theta)*sin(phi))-(2*u1*theta_dot*phi_dot*sin(theta)*sin(phi))+(u1*(((theta_dot*theta_dot))-((phi_dot*phi_dot)))*cos(theta)*cos(phi))+v3];


m1i=inv(m1);

m3=m1i*m2;

u1_ddot= m3(1,1);
u2=m3(2,1);
u3=m3(3,1);

== matlab function Feedback_Linearization/Enabled Subsystem/Quadcopter /Quadcopter Dynamics ==
  data: u1 input; xdd output; u2 input; u3 input; u4 input; ydd output; zdd output; phidd output; thetadd output; psidd output; phi input; theta input
function [xdd,ydd,zdd,phidd,thetadd,psidd] = fcn(u1,u2,u3,u4,phi,theta)

xdd=u1*sin(theta);
ydd=-u1*sin(phi);
zdd=(u1*cos(phi)*cos(theta))-9.81;
phidd=u2;
thetadd=u3;
psidd=u4;

== matlab function Feedback_Linearization/Enabled Subsystem1/FL Controller4/MATLAB Function ==
  data: v1 input; u1_ddot output; v2 input; v3 input; phi input; theta input; theta_dot input; phi_dot input; u1 input; u1_dot input; u2 output; u3 output
function [u1_ddot,u2,u3] = fcn(v1,v2,v3,phi,theta,theta_dot,phi_dot,u1,u1_dot)

m1=[[sin(theta),0,(u1)*cos(theta)];
    [-sin(phi),(-u1*cos(phi)),0];
    [(cos(theta)*cos(phi)),(-u1*cos(theta)*sin(phi)),(-u1*sin(theta)*cos(phi))]];


m2=[(-2*u1_dot*theta_dot*cos(theta))+(u1*((theta_dot*theta_dot))*sin(theta))+v1;
    (2*u1_dot*phi_dot*cos(phi))-(u1*((phi_dot*phi_dot))*sin(phi))+v2;
    (2*u1_dot*theta_dot*sin(theta)*cos(phi))+(2*u1_dot*phi_dot*cos(theta)*sin(phi))-(2*u1*theta_dot*phi_dot*sin(theta)*sin(phi))+(u1*(((theta_dot*theta_dot))-((phi_dot*phi_dot)))*cos(theta)*cos(phi))+v3];


m1i=inv(m1);

m3=m1i*m2;

u1_ddot= m3(1,1);
u2=m3(2,1);
u3=m3(3,1);

== matlab function Feedback_Linearization/Enabled Subsystem1/Quadcopter 2/Quadcopter Dynamics ==
  data: u1 input; xdd output; u2 input; u3 input; u4 input; ydd output; zdd output; phidd output; thetadd output; psidd output; phi input; theta input
function [xdd,ydd,zdd,phidd,thetadd,psidd] = fcn(u1,u2,u3,u4,phi,theta)

xdd=u1*sin(theta);
ydd=-u1*sin(phi);
zdd=(u1*cos(phi)*cos(theta))-9.81;
phidd=u2;
thetadd=u3;
psidd=u4;
